simulink model "unicycle_b_point"  (R2025b)
settings: Solver=ode5  StartTime=0.0  StopTime=40  FixedStep=1e-3  MaxStep=0.01  RelTol=1e-3
libraries: dspsigops x1
settings Model: Creator=Cris  LastModifiedBy=Cris
settings DebuggingCC: UnderspecifiedInitializationDetection=Classic  MergeDetectMultiDrivingBlocksExec=none
settings ModelReferenceCC: PropagateSignalLabelsOutOfModel=off

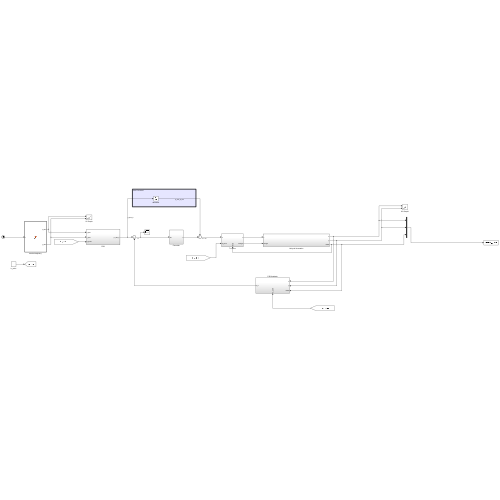
[thumbnail: Simulink's stored preview of the top-level diagram]
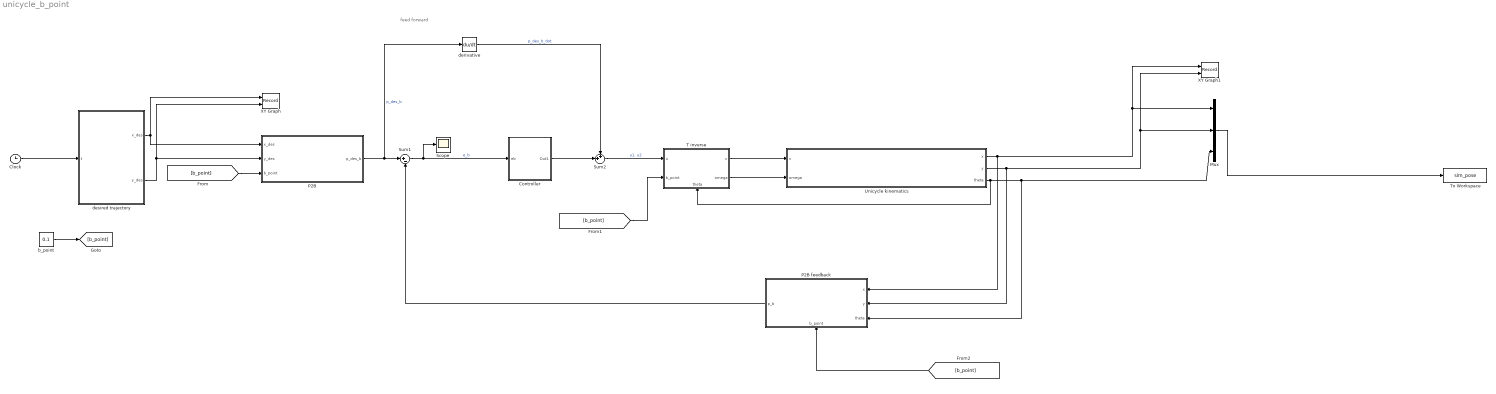
== system unicycle_b_point ==
  note: feed forward
  Clock : Clock
  Controller : Subsystem
  Mux : Mux  Inputs=3
  P2B : Subsystem
  P2B feedback : Subsystem
      settings: PortSchema="{\"entries\":[{\"content\":{\"sides\":[{\"content\":{\"connectorIds\":[\"In1\",\"In2\",\"In3\"]},\"type\":\"ConnectorPlacement.EquallySpacedRectSide\",\"uuid\":\"f90c83b3-4884-4b15-8db2-3ad54e7fbcd2\"},{\"content\":{\"connectorIds\":[\"Out1\"],\"side\":\"RIGHT\"},\"type\":\"ConnectorPlacement.EquallySpacedRectSide\",\"uuid\":\"0e9bf0d6-0706-43e1-b116-579d07e0d7a9\"},{\"content\":{\"side\":\"TOP\"},\"type\":\"ConnectorPlacement.EquallySpacedRectSide\",\"uuid\":\"aa0be909-bf73-4da0-8969-0ac18978c817\"},{\"content\":{\"connectorIds\":[\"In4\"],\"side\":\"BOTTOM\"},\"type\":\"ConnectorPlacement.EquallySpacedRectSide\",\"uuid\":\"2cd6bdb7-80fd-4c63-a9e6-03da628bdfe9\"}]},\"type\":\"ConnectorPlacement.EquallySpacedConnector\",\"uuid\":\"d66b1899-20f1-4272-bfb5-fa44cb619962\"}],\"packageUris\":[\"http://schema.mathworks.com/mf0/Connector/R2020b\"],\"version\":\"1.0\"}"
  Scope : Scope
      settings: ActiveDisplayYMinimum=-2.3496580332786578E+11  ActiveDisplayYMaximum=2.1146922300504998E+12
  Sum1 : Sum  Inputs=|+-
  Sum2 : Sum  Inputs=++|
  T inverse : Subsystem
      settings: PortSchema="{\"entries\":[{\"content\":{\"sides\":[{\"content\":{\"connectorIds\":[\"In1\",\"In2\"]},\"type\":\"ConnectorPlacement.EquallySpacedRectSide\",\"uuid\":\"6a572e67-edde-4e1b-8365-e17ad9f48dde\"},{\"content\":{\"connectorIds\":[\"Out1\",\"Out2\"],\"side\":\"RIGHT\"},\"type\":\"ConnectorPlacement.EquallySpacedRectSide\",\"uuid\":\"eef3ef4a-e0db-4110-95fe-7b093a8263df\"},{\"content\":{\"side\":\"TOP\"},\"type\":\"ConnectorPlacement.EquallySpacedRectSide\",\"uuid\":\"36409ed0-e85a-4572-922e-f9880c3e6c77\"},{\"content\":{\"connectorIds\":[\"In3\"],\"side\":\"BOTTOM\"},\"type\":\"ConnectorPlacement.EquallySpacedRectSide\",\"uuid\":\"15817285-2ec7-4fec-a753-9fcf1bcbe7f7\"}]},\"type\":\"ConnectorPlacement.EquallySpacedConnector\",\"uuid\":\"7cf4f3ea-e25c-438d-a1f8-97a6ff8f9133\"}],\"packageUris\":[\"http://schema.mathworks.com/mf0/Connector/R2020b\"],\"version\":\"1.0\"}"
  To Workspace : ToWorkspace  VariableName=sim_pose  SaveFormat=Timeseries  SampleTime=-1
  Unicycle kinematics : Subsystem
  XY Graph : Record  NumPorts=2.0  FileSettingsInternal="{\"entries\":[{\"content\":{\"excelSettings\":{\"content\":{},\"type\":\"Streamout.ExcelSettings\"},\"parquetSettings\":{\"content\":{},\"type\":\"Streamout.ParquetSettings\"}},\"type\":\"Streamout.FileSettingStorage\",\"uuid\":\"\"}],\"packageUris\":[\"http:\\/\\/schema.mathworks.com\\/mf0\\/streamout_blocks\\/R2020a\"],\"version\":\"1.0\"}"  FrameSettings=[0, 0]  Layout=[1 1]  SignalsInternal="{\"entries\":[{\"content\":{\"signals\":[{\"content\":{\"blockPath\":[],\"dimensions\":[1],\"domain\":\"\",\"lineColor\":\"#a2142f\",\"plots\":[ 1 ],\"port\":1,\"sid\":[\"\"],\"signalID\":1,\"signalName\":\"desired trajectory:1\"},\"type\":\"RecordBlkView.Signal\",\"uuid\":\"\"},{\"content\":{\"blockPath\":[],\"dimensions\":[1],\"domain\":\"\",\"lineColor\":\"#139fff\",\"plots\":[ 1 ],\"port\":2,\"sid\":[\"\"],\"signalID\":2,\"signalName\":\"desired trajectory:2\"},\"type\":\"RecordBlkView.Signal\",\"uuid\":\"\"}]},\"type\":\"RecordBlkView.InputSignals\",\"uuid\":\"\"}],\"packageUris\":[\"http:\\/\\/schema.mathworks.com\\/mf0\\/streamout_blocks\\/R2020a\"],\"version\":\"1.0\"}"  VisualizationBindings="{\"xyplotplugin\":{\"info\":[{\"series\":[{\"bindingParametersList\":[{\"parameter\":\"X-Axis\",\"signalID\":1,\"signalName\":\"desired trajectory:1\"},{\"parameter\":\"Y-Axis\",\"signalID\":2,\"signalName\":\"desired trajectory:2\"}],\"seriesID\":0}],\"subplotID\":1}]}}"  CompatibilityTag=XY
  XY Graph1 : Record  NumPorts=2.0  FileSettingsInternal="{\"entries\":[{\"content\":{\"excelSettings\":{\"content\":{},\"type\":\"Streamout.ExcelSettings\"},\"parquetSettings\":{\"content\":{},\"type\":\"Streamout.ParquetSettings\"}},\"type\":\"Streamout.FileSettingStorage\",\"uuid\":\"\"}],\"packageUris\":[\"http:\\/\\/schema.mathworks.com\\/mf0\\/streamout_blocks\\/R2020a\"],\"version\":\"1.0\"}"  FrameSettings=[0, 0]  Layout=[1 1]  SignalsInternal="{\"entries\":[{\"content\":{\"signals\":[{\"content\":{\"blockPath\":[],\"dimensions\":[1],\"domain\":\"\",\"lineColor\":\"#a2142f\",\"plots\":[ 1 ],\"port\":1,\"sid\":[\"\"],\"signalID\":1,\"signalName\":\"Unicycle kinematics:1\"},\"type\":\"RecordBlkView.Signal\",\"uuid\":\"\"},{\"content\":{\"blockPath\":[],\"dimensions\":[1],\"domain\":\"\",\"lineColor\":\"#139fff\",\"plots\":[ 1 ],\"port\":2,\"sid\":[\"\"],\"signalID\":2,\"signalName\":\"Unicycle kinematics:2\"},\"type\":\"RecordBlkView.Signal\",\"uuid\":\"\"}]},\"type\":\"RecordBlkView.InputSignals\",\"uuid\":\"\"}],\"packageUris\":[\"http:\\/\\/schema.mathworks.com\\/mf0\\/streamout_blocks\\/R2020a\"],\"version\":\"1.0\"}"  VisualizationBindings="{\"xyplotplugin\":{\"info\":[{\"series\":[{\"bindingParametersList\":[{\"parameter\":\"X-Axis\",\"signalID\":1,\"signalName\":\"Unicycle kinematics:1\"},{\"parameter\":\"Y-Axis\",\"signalID\":2,\"signalName\":\"Unicycle kinematics:2\"}],\"seriesID\":0}],\"subplotID\":1}]}}"  CompatibilityTag=XY
  b_point : Constant  Value=0.1
  derivative : Derivative
  desired trajectory : MATLAB Function  TreatAsAtomicUnit=on
  wires:
  Unicycle kinematics/1(x) -> XY Graph1/1, Mux/1, P2B feedback/1(x)
  Unicycle kinematics/2(y) -> P2B feedback/2(y), XY Graph1/2, Mux/2
  Unicycle kinematics/3(theta) -> T inverse/3(theta), P2B feedback/3(theta), Mux/3
  desired trajectory/1(x_des) -> P2B/1(x_des), XY Graph/1
  desired trajectory/2(y_des) -> P2B/2(y_des), XY Graph/2
  Clock/1 -> desired trajectory/1(t)
  Mux/1 -> To Workspace/1
  derivative/1 -> Sum2/1  "p_des_b_dot"
  P2B/1(p_des_b) -> derivative/1, Sum1/1  "p_des_b"
  Sum1/1 -> Scope/1, Controller/1(eb)  "e_b"
  Controller/1(Out1) -> Sum2/2
  Sum2/1 -> T inverse/1(u)  "u1, u2"
  b_point/1 -> [b_point]
  [b_point] -> P2B/3(b_point)
  [b_point] -> T inverse/2(b_point)
  T inverse/1(v) -> Unicycle kinematics/1(v)
  T inverse/2(omega) -> Unicycle kinematics/2(omega)
  [b_point] -> P2B feedback/4(b_point)
  P2B feedback/1(p_b) -> Sum1/2

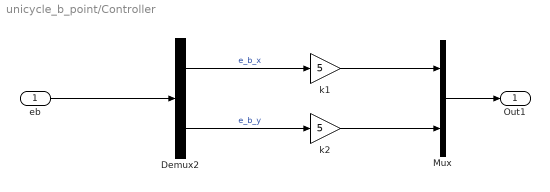
== system unicycle_b_point/Controller ==
  eb : Inport
  Demux2 : Demux  Outputs=2
  Mux : Mux  Inputs=2
  k1 : Gain  Gain=5
  k2 : Gain  Gain=5
  Out1 : Outport
  wires:
  k2/1 -> Mux/2
  Mux/1 -> Out1/1
  Demux2/1 -> k1/1  "e_b_x"
  k1/1 -> Mux/1
  Demux2/2 -> k2/1  "e_b_y"
  eb/1 -> Demux2/1

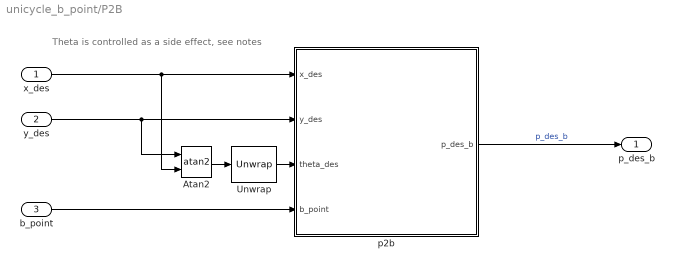
== system unicycle_b_point/P2B ==
  note: Theta is controlled as a side effect, see notes
  x_des : Inport
  y_des : Inport  Port=2
  b_point : Inport  Port=3
  Atan2 : Trigonometry  Operator=atan2
  Unwrap : dspsigops/Unwrap  tol=pi  InputProcessing=Columns as channels (frame based)  running=off
  p2b : MATLAB Function  TreatAsAtomicUnit=on
  p_des_b : Outport
  wires:
  p2b/1(p_des_b) -> p_des_b/1  "p_des_b"
  x_des/1 -> Atan2/2, p2b/1(x_des)
  y_des/1 -> Atan2/1, p2b/2(y_des)
  Atan2/1 -> Unwrap/1
  Unwrap/1 -> p2b/3(theta_des)
  b_point/1 -> p2b/4(b_point)

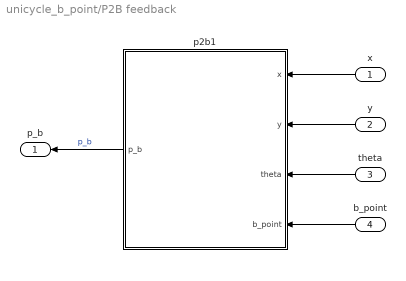
== system unicycle_b_point/P2B feedback ==
  x : Inport
  y : Inport  Port=2
  theta : Inport  Port=3
  b_point : Inport  Port=4
  p2b1 : MATLAB Function  TreatAsAtomicUnit=on
  p_b : Outport
  wires:
  x/1 -> p2b1/1(x)
  y/1 -> p2b1/2(y)
  theta/1 -> p2b1/3(theta)
  b_point/1 -> p2b1/4(b_point)
  p2b1/1(p_b) -> p_b/1  "p_b"

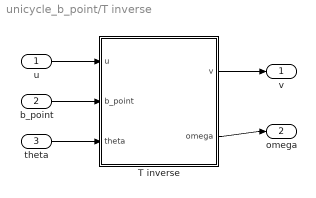
== system unicycle_b_point/T inverse ==
  u : Inport
  b_point : Inport  Port=2
  theta : Inport  Port=3
  T inverse : MATLAB Function  TreatAsAtomicUnit=on
  v : Outport
  omega : Outport  Port=2
  wires:
  u/1 -> T inverse/1(u)
  theta/1 -> T inverse/3(theta)
  b_point/1 -> T inverse/2(b_point)
  T inverse/1(v) -> v/1
  T inverse/2(omega) -> omega/1

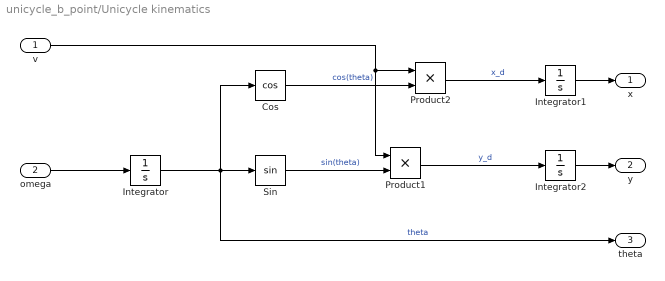
== system unicycle_b_point/Unicycle kinematics ==
  v : Inport
  omega : Inport  Port=2
  Cos : Trigonometry  Operator=cos
  Integrator : Integrator
  Integrator1 : Integrator
  Integrator2 : Integrator
  Product1 : Product
  Product2 : Product
  Sin : Trigonometry
  x : Outport
  y : Outport  Port=2
  theta : Outport  Port=3
  wires:
  omega/1 -> Integrator/1
  Integrator/1 -> theta/1, Cos/1, Sin/1  "theta"
  Cos/1 -> Product2/2  "cos(theta)"
  Sin/1 -> Product1/2  "sin(theta)"
  v/1 -> Product2/1, Product1/1
  Integrator1/1 -> x/1
  Product2/1 -> Integrator1/1  "x_d"
  Integrator2/1 -> y/1
  Product1/1 -> Integrator2/1  "y_d"

== matlab function unicycle_b_point/P2B feedback/p2b1 ==
  data: x input; y input; theta input; p_b output; b_point input
function p_b = fcn(x, y, theta, b_point)

x_b = x + b_point * cos(theta);
y_b = y + b_point * sin(theta);

p_b = [x_b; y_b];

== matlab function unicycle_b_point/P2B/p2b ==
  data: x_des input; y_des input; theta_des input; p_des_b output; b_point input
function p_des_b = fcn(x_des, y_des, theta_des,  b_point)

x_b = x_des + b_point * cos(theta_des);
y_b = y_des + b_point * sin(theta_des);

p_des_b = [x_b; y_b];

== matlab function unicycle_b_point/desired trajectory ==
  data: t input; x_des output; y_des output
function [x_des, y_des] = fcn(t)

% % configurable:
% radius = 5;
% omega_des = 0.2;
% 
% % desired trajectory
% x_des = -radius*cos(omega_des*t);
% y_des = -radius*sin(omega_des*t);


% % configurable:
% radius = 10;
% omega_des = 0.5;
% 
% % desired trajectory
% x_des = radius*cos(omega_des*t);
% y_des = radius*sin(omega_des*t);
% 


if t <= 10
    x_des = 10+t;
    y_des = 10;
elseif  t <= 20
    x_des = 20;
    y_des = 0+t;
elseif  t <= 30
    x_des = 40-t;
    y_des = 20;
elseif  t <= 40
    x_des = 10;
    y_des = 50-t;
else
    x_des = 100;
    y_des = 100;
end

== matlab function unicycle_b_point/T inverse/T inverse ==
  data: u input size=2; b_point input size=1; v output size=1; omega output size=1; theta input size=1
function [v, omega] = fcn(u, b_point, theta)

% define matrix T inverse
T_inv = (1/b_point)*[b_point*cos(theta), b_point*sin(theta);
    -sin(theta), cos(theta)];

% do calculation
res = T_inv * u;

% assign output
v = res(1, 1);
omega = res(2, 1);
